simulink model "flexy_air_blank"  (R2020a)
settings: Solver=FixedStepAuto  StartTime=0.0  StopTime=Inf  FixedStep=Ts  RelTol=1e-3
libraries: flexy_air_lib x1
settings Model: EnablePacing=on  Creator=MK  LastModifiedBy=MK

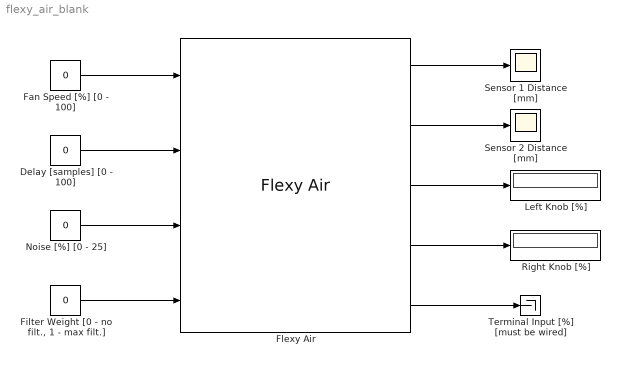
== system flexy_air_blank ==
  Delay [samples] [0 - 100] : Constant  Value=0
  Fan Speed [%] [0 - 100] : Constant  Value=0
  "Filter Weight [0 - no filt., 1 - max filt.]" : Constant  Value=0
  Flexy Air : flexy_air_lib/Flexy Air  SystemSampleTime=-1  Latency=0  AutoFrameSizeCalculation=off
  "Left Knob [%] " : Display
  Noise [%] [0 - 25] : Constant  Value=0
  "Right Knob [%] " : Display
  Sensor 1 Distance [mm] : Scope
  Sensor 2 Distance [mm] : Scope
  Terminal Input [%] [must be wired] : Terminator
  wires:
  Fan Speed [%] [0 - 100]/1 -> Flexy Air/1
  Delay [samples] [0 - 100]/1 -> Flexy Air/2
  Noise [%] [0 - 25]/1 -> Flexy Air/3
  "Filter Weight [0 - no filt., 1 - max filt.]"/1 -> Flexy Air/4
  Flexy Air/1 -> Sensor 1 Distance [mm]/1
  Flexy Air/2 -> Sensor 2 Distance [mm]/1
  Flexy Air/3 -> "Left Knob [%] "/1
  Flexy Air/4 -> "Right Knob [%] "/1
  Flexy Air/5 -> Terminal Input [%] [must be wired]/1
